simulink model "simula"  (R2018a)
settings: Solver=VariableStepAuto  StartTime=0.0  StopTime=inf  RelTol=1e-3
values from neighbouring files (symbols this model uses):
  Qn = 1e-5*eye(4)    [main.m]
  Qn_euler = [0.01 0 0 0 0 0 ... (first row only)    [main.m]
  Qn_v2 = 1e-5*eye(7)    [main.m]
  Rn = 0.71e-3*eye(6)    [main.m]
  Rn_euler = 0.20*eye(3)    [main.m]
  Ts = 1/25    (= 0.04)    [main.m]
libraries: aerolibutil x2, sharedutil x1
settings Model: Creator=marcus  LastModifiedBy=marcus

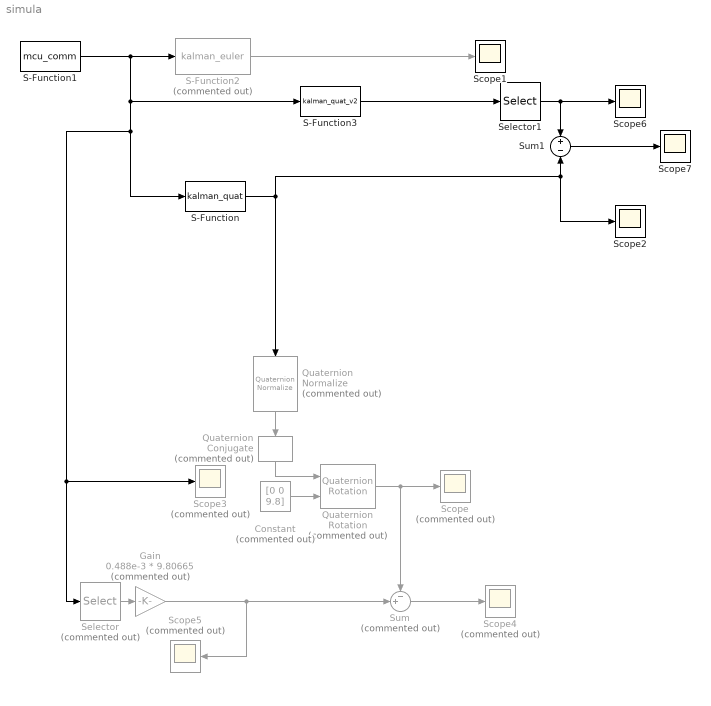
== system simula ==
  Constant : Constant  Commented=on  Value=[0 0 9.8]
  Gain : Gain  Commented=on  Gain=0.488e-3 * 9.80665
  Quaternion Conjugate : aerolibutil/Quaternion Conjugate  Commented=on
      settings: SourceProductName=Aerospace Blockset  SourceProductBaseCode=AE
  Quaternion Normalize : sharedutil/Quaternion Normalize  Commented=on  aMode=aMode
      settings: SourceProductName=Aerospace Blockset  SourceProductBaseCode=AE
  Quaternion Rotation : aerolibutil/Quaternion Rotation  Commented=on
  S-Function : S-Function  FunctionName=kalman_quat  Parameters=Ts,Qn,Rn  SFunctionDeploymentMode=off  EnableBusSupport=off
  S-Function1 : S-Function  FunctionName=mcu_comm  Parameters=Ts  SFunctionDeploymentMode=off  EnableBusSupport=off
  S-Function2 : S-Function  Commented=on  FunctionName=kalman_euler  Parameters=Ts,Qn_euler,Rn_euler  SFunctionDeploymentMode=off  EnableBusSupport=off
  S-Function3 : S-Function  FunctionName=kalman_quat_v2  Parameters=Ts,Qn_v2,Rn  SFunctionDeploymentMode=off  EnableBusSupport=off
  Scope{,3..5} (4 alike) : Scope  Commented=on
  Scope{1..2,6..7} (4 alike) : Scope
  Selector : Selector  Commented=on  InputPortWidth=9  IndexOptions=Index vector (dialog)  Indices=[1 2 3]  OutputSizes=1
  Selector1 : Selector  InputPortWidth=7  IndexOptions=Index vector (dialog)  Indices=1:4  OutputSizes=1
  Sum : Sum  Commented=on  Inputs=-+|
  Sum1 : Sum  Inputs=+-
  wires:
  S-Function/1 -> Sum1/2, Scope2/1, Quaternion Normalize/1
  S-Function2/1 -> Scope1/1
  S-Function1/1 -> S-Function/1, Scope3/1, Selector/1, S-Function3/1, S-Function2/1
  Quaternion Rotation/1 -> Sum/1, Scope/1
  Selector/1 -> Gain/1
  Constant/1 -> Quaternion Rotation/2
  Gain/1 -> Scope5/1, Sum/2
  Sum/1 -> Scope4/1
  Quaternion Conjugate/1 -> Quaternion Rotation/1
  Quaternion Normalize/1 -> Quaternion Conjugate/1
  S-Function3/1 -> Selector1/1
  Selector1/1 -> Sum1/1, Scope6/1
  Sum1/1 -> Scope7/1
